simulink model "OES"  (R2018b)
settings: configuration reference "Configuration" (kept outside this file)
undefined symbols (not defined in the file): CON, sat, sats
settings Model: Creator=Ethan  LastModifiedBy=Ethan
settings ConfigSetRef: SourceLocation=Base Workspace

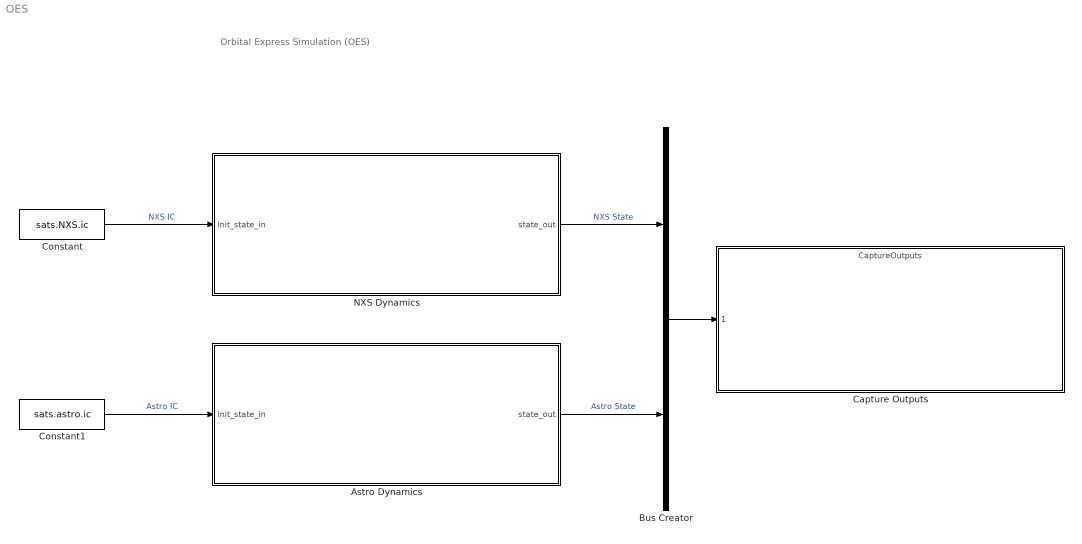
== system OES ==
  note: Orbital Express Simulation (OES)
  Astro Dynamics : Subsystem  Variant=on
  Bus Creator : BusCreator  Inputs=2  OutDataTypeStr=Bus: Bus_outputs  NonVirtualBus=on
      settings: InheritFromInputs=off
  Capture Outputs : ModelReference  ModelNameDialog=CaptureOutputs.slx  ParameterArgumentNames=CON  ParameterArgumentValues=CON  UsingDefaultArgumentValue=0  SimulationMode=Normal  ModelReferenceVersion=1.39
  Constant : Constant  Value=sats.NXS.ic  OutDataTypeStr=Bus: Bus_state
  Constant1 : Constant  Value=sats.astro.ic  OutDataTypeStr=Bus: Bus_state
  NXS Dynamics : Subsystem  Variant=on
  wires:
  Constant/1 -> NXS Dynamics/1(init_state_in)  "NXS IC"
  Constant1/1 -> Astro Dynamics/1(init_state_in)  "Astro IC"
  Astro Dynamics/1(state_out) -> Bus Creator/2  "Astro State"
  NXS Dynamics/1(state_out) -> Bus Creator/1  "NXS State"
  Bus Creator/1 -> Capture Outputs/1

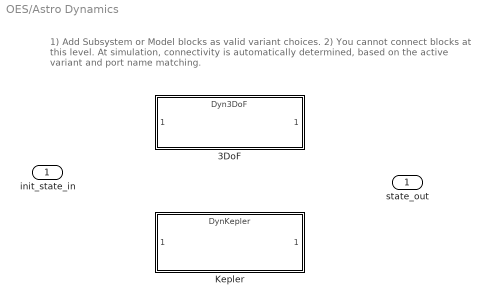
== system OES/Astro Dynamics ==
  note: 1) Add Subsystem or Model blocks as valid variant choices.
      | 2) You cannot connect blocks at this level. At simulation, connectivity is automatically
      | determined, based on the active variant and port name matching.
  init_state_in : Inport
  3DoF : ModelReference  DisableCoverage=on  ModelNameDialog=Dyn3DoF.slx  ParameterArgumentNames=CON,sat  ParameterArgumentValues=CON,sats.astro  UsingDefaultArgumentValue=0,0  VariantControl=Dyn3DoF_variant  ModelReferenceVersion=1.53
  Kepler : ModelReference  ModelNameDialog=DynKepler.slx  ParameterArgumentNames=CON  ParameterArgumentValues=CON  UsingDefaultArgumentValue=0  SimulationMode=Normal  VariantControl=Kepler_variant  ModelReferenceVersion=1.72
  state_out : Outport

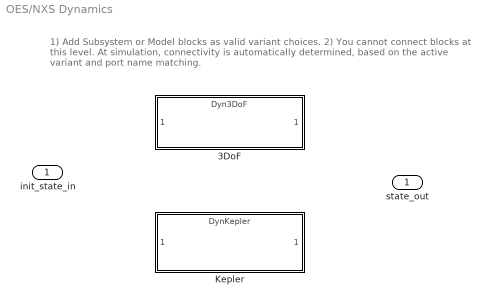
== system OES/NXS Dynamics ==
  note: 1) Add Subsystem or Model blocks as valid variant choices.
      | 2) You cannot connect blocks at this level. At simulation, connectivity is automatically
      | determined, based on the active variant and port name matching.
  init_state_in : Inport
  3DoF : ModelReference  DisableCoverage=on  ModelNameDialog=Dyn3DoF.slx  ParameterArgumentNames=CON,sat  ParameterArgumentValues=CON,sats.NXS  UsingDefaultArgumentValue=0,0  SimulationMode=Normal  VariantControl=Dyn3DoF_variant  ModelReferenceVersion=1.53
  Kepler : ModelReference  ModelNameDialog=DynKepler.slx  ParameterArgumentNames=CON  ParameterArgumentValues=CON  UsingDefaultArgumentValue=0  VariantControl=Kepler_variant  ModelReferenceVersion=1.72
  state_out : Outport
